simulink model "SkywalkerX8_SensorSuite"  (R2018a)
settings: Solver=FixedStepAuto  StartTime=0.0  StopTime=SkywalkerX8.Sensors.TestProfile.Time(end)  FixedStep=SkywalkerX8.Sensors.TestProfile.Time(2)/100  RelTol=1e-3
undefined symbols (not defined in the file): SkywalkerX8
libraries: sensors x7
settings Model: Creator=David  LastModifiedBy=David

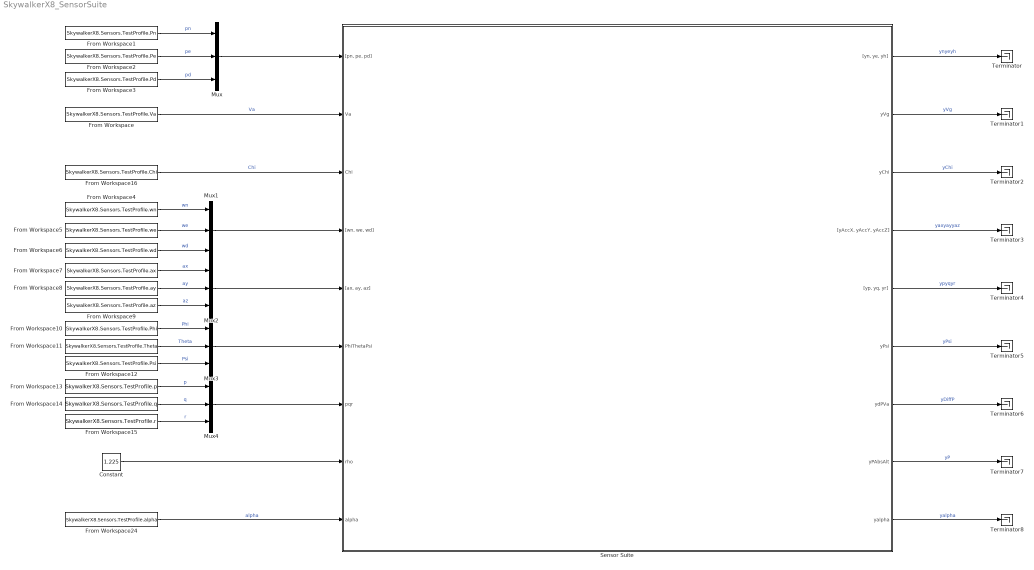
== system SkywalkerX8_SensorSuite ==
  Constant : Constant  Value=1.225
  From Workspace : FromWorkspace  VariableName=SkywalkerX8.Sensors.TestProfile.Va  SampleTime=SkywalkerX8.Sensors.TestProfile.Time(2)  Interpolate=off  OutputAfterFinalValue=Holding final value
  From Workspace1 : FromWorkspace  VariableName=SkywalkerX8.Sensors.TestProfile.Pn  SampleTime=SkywalkerX8.Sensors.TestProfile.Time(2)  Interpolate=off  OutputAfterFinalValue=Holding final value
  From Workspace10 : FromWorkspace  VariableName=SkywalkerX8.Sensors.TestProfile.Phi  SampleTime=SkywalkerX8.Sensors.TestProfile.Time(2)  Interpolate=off  OutputAfterFinalValue=Holding final value
  From Workspace11 : FromWorkspace  VariableName=SkywalkerX8.Sensors.TestProfile.Theta  SampleTime=SkywalkerX8.Sensors.TestProfile.Time(2)  Interpolate=off  OutputAfterFinalValue=Holding final value
  From Workspace12 : FromWorkspace  VariableName=SkywalkerX8.Sensors.TestProfile.Psi  SampleTime=SkywalkerX8.Sensors.TestProfile.Time(2)  Interpolate=off  OutputAfterFinalValue=Holding final value
  From Workspace13 : FromWorkspace  VariableName=SkywalkerX8.Sensors.TestProfile.p  SampleTime=SkywalkerX8.Sensors.TestProfile.Time(2)  Interpolate=off  OutputAfterFinalValue=Holding final value
  From Workspace14 : FromWorkspace  VariableName=SkywalkerX8.Sensors.TestProfile.q  SampleTime=SkywalkerX8.Sensors.TestProfile.Time(2)  Interpolate=off  OutputAfterFinalValue=Holding final value
  From Workspace15 : FromWorkspace  VariableName=SkywalkerX8.Sensors.TestProfile.r  SampleTime=SkywalkerX8.Sensors.TestProfile.Time(2)  Interpolate=off  OutputAfterFinalValue=Holding final value
  From Workspace16 : FromWorkspace  VariableName=SkywalkerX8.Sensors.TestProfile.Chi  SampleTime=SkywalkerX8.Sensors.TestProfile.Time(2)  Interpolate=off  OutputAfterFinalValue=Holding final value
  From Workspace2 : FromWorkspace  VariableName=SkywalkerX8.Sensors.TestProfile.Pe  SampleTime=SkywalkerX8.Sensors.TestProfile.Time(2)  Interpolate=off  OutputAfterFinalValue=Holding final value
  From Workspace24 : FromWorkspace  VariableName=SkywalkerX8.Sensors.TestProfile.alpha  SampleTime=SkywalkerX8.Sensors.TestProfile.Time(2)  Interpolate=off  OutputAfterFinalValue=Holding final value
  From Workspace3 : FromWorkspace  VariableName=SkywalkerX8.Sensors.TestProfile.Pd  SampleTime=SkywalkerX8.Sensors.TestProfile.Time(2)  Interpolate=off  OutputAfterFinalValue=Holding final value
  From Workspace4 : FromWorkspace  VariableName=SkywalkerX8.Sensors.TestProfile.wn  SampleTime=SkywalkerX8.Sensors.TestProfile.Time(2)  Interpolate=off  OutputAfterFinalValue=Holding final value
  From Workspace5 : FromWorkspace  VariableName=SkywalkerX8.Sensors.TestProfile.we  SampleTime=SkywalkerX8.Sensors.TestProfile.Time(2)  Interpolate=off  OutputAfterFinalValue=Holding final value
  From Workspace6 : FromWorkspace  VariableName=SkywalkerX8.Sensors.TestProfile.wd  SampleTime=SkywalkerX8.Sensors.TestProfile.Time(2)  Interpolate=off  OutputAfterFinalValue=Holding final value
  From Workspace7 : FromWorkspace  VariableName=SkywalkerX8.Sensors.TestProfile.ax  SampleTime=SkywalkerX8.Sensors.TestProfile.Time(2)  Interpolate=off  OutputAfterFinalValue=Holding final value
  From Workspace8 : FromWorkspace  VariableName=SkywalkerX8.Sensors.TestProfile.ay  SampleTime=SkywalkerX8.Sensors.TestProfile.Time(2)  Interpolate=off  OutputAfterFinalValue=Holding final value
  From Workspace9 : FromWorkspace  VariableName=SkywalkerX8.Sensors.TestProfile.az  SampleTime=SkywalkerX8.Sensors.TestProfile.Time(2)  Interpolate=off  OutputAfterFinalValue=Holding final value
  Mux{,1..4} (5 alike) : Mux  Inputs=3
  Sensor Suite : Subsystem
      mask Display:
      | image('telemetry.jpg')
      | 
      | color('cyan')
      | 
      | port_label('input', 1, '[p_N, p_E, p_D] (m)', 'texMode', 'On')
      | port_label('input', 2, 'V_a (m/s)', 'texMode', 'On')
      | port_label('input', 3, '\chi (rad)', 'texMode', 'On')
      | port_label('input', 4, '[w_N, w_E, w_D] (m/s)', 'texMode', 'On')
      | port_label('input', 5, '{\bfa_{inertial}} (m/s^2)', 'texMode', 'on')
      | port_label('input', 6, '[\phi, \theta, \psi] (rad)', 'texMode', 'on')
      | port_label('input', 7, '{\bf\omega_b} (rad/s)', 'texMode', 'on')
      | port_label('input', 8, '\rho (kg/m^3)', 'texMode', 'on')
      | port_label('input', 9, '\alpha (rad)', 'texMode', 'on')
      | 
      | port_label('output', 1, '[y_{GPS_N}, y_{GPS_E}, y_{GPS_h}] (m)', 'texMode', 'On')
      | port_label('output', 2, 'y_{GPS_{Vg}} (m/s)', 'texMode', 'On')
      | port_label('output', 3, 'y_{GPS_{\chi}} (rad)', 'texMode', 'On')
      | port_label('output', 4, '[y_{accel_x}, y_{accel_y}, y_{accel_z}] (m/s^2)', 'texMode', 'on')
      | port_label('output', 5, '[y_p, y_q, y_r] (rad/s)', 'texMode', 'on')
      | port_label('output', 6, 'y_{\psi} (rad)', 'texMode', 'on')
      | port_label('output', 7, 'y_{\DeltaP_{V_a}} (Pa)', 'texMode', 'on')
      | port_label('output', 8, 'y_{P_{abs}} (Pa)', 'texMode', 'on')
      | port_label('output', 9, 'y_\alpha (rad)', 'texMode', 'on')
  Terminator{,1..8} (9 alike) : Terminator
  wires:
  Sensor Suite/1("[yn, ye, yh]") -> Terminator/1  "ynyeyh"
  Sensor Suite/2(yVg) -> Terminator1/1  "yVg"
  Sensor Suite/3(yChi) -> Terminator2/1  "yChi"
  Sensor Suite/4("[yAccX, yAccY, yAccZ]") -> Terminator3/1  "yaxyayyaz"
  Sensor Suite/5("[yp, yq, yr]") -> Terminator4/1  "ypyqyr"
  Sensor Suite/6(yPsi) -> Terminator5/1  "yPsi"
  Sensor Suite/7(ydPVa) -> Terminator6/1  "yDiffP"
  Sensor Suite/8(yPAbsAlt) -> Terminator7/1  "yP"
  Mux3/1 -> Sensor Suite/6(PhiThetaPsi)
  Mux/1 -> Sensor Suite/1("[pn, pe, pd]")
  Mux4/1 -> Sensor Suite/7(pqr)
  Mux1/1 -> Sensor Suite/4("[wn, we, wd]")
  From Workspace3/1 -> Mux/3  "pd"
  From Workspace6/1 -> Mux1/3  "wd"
  From Workspace9/1 -> Mux2/3  "az"
  Constant/1 -> Sensor Suite/8(rho)
  From Workspace1/1 -> Mux/1  "pn"
  From Workspace11/1 -> Mux3/2  "Theta"
  From Workspace7/1 -> Mux2/1  "ax"
  From Workspace10/1 -> Mux3/1  "Phi"
  From Workspace4/1 -> Mux1/1  "wn"
  From Workspace8/1 -> Mux2/2  "ay"
  From Workspace12/1 -> Mux3/3  "Psi"
  From Workspace2/1 -> Mux/2  "pe"
  From Workspace14/1 -> Mux4/2  "q"
  From Workspace5/1 -> Mux1/2  "we"
  From Workspace/1 -> Sensor Suite/2(Va)  "Va"
  From Workspace15/1 -> Mux4/3  "r"
  Mux2/1 -> Sensor Suite/5("[ax, ay, az]")
  From Workspace13/1 -> Mux4/1  "p"
  From Workspace24/1 -> Sensor Suite/9(alpha)  "alpha"
  Sensor Suite/9(yalpha) -> Terminator8/1  "yalpha"
  From Workspace16/1 -> Sensor Suite/3(Chi)  "Chi"

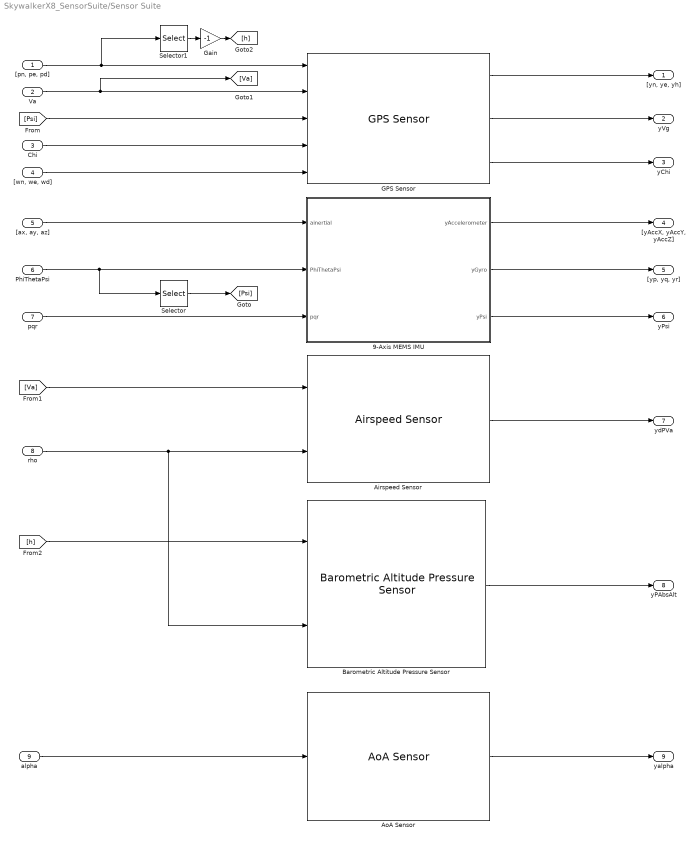
== system SkywalkerX8_SensorSuite/Sensor Suite ==
  "[pn, pe, pd]" : Inport
  Va : Inport  Port=2
  Chi : Inport  Port=3
  "[wn, we, wd]" : Inport  Port=4
  "[ax, ay, az]" : Inport  Port=5
  PhiThetaPsi : Inport  Port=6
  pqr : Inport  Port=7
  rho : Inport  Port=8
  alpha : Inport  Port=9
  9-Axis MEMS IMU : Subsystem
      mask Display:
      | image('VNAV_IMU.jpg')
      | 
      | color('green')
      | 
      | port_label('input', 1, '{\bfa_{inertial}} (m/s^2)', 'texMode', 'on')
      | port_label('input', 2, '[\phi, \theta, \psi] (rad)', 'texMode', 'on')
      | port_label('input', 3, '{\bf\omega_b} (rad/s)', 'texMode', 'on')
      | 
      | port_label('output', 1, '[y_{accel_x}, y_{accel_y}, y_{accel_z}] (m/s^2)', 'texMode', 'on')
      | port_label('output', 2, '[y_p, y_q, y_r] (rad/s)', 'texMode', 'on')
      | port_label('output', 3, 'y_{\psi} (rad)', 'texMode', 'on')
  Airspeed Sensor : sensors/Airspeed Sensor  SampleTime=SkywalkerX8.Sensors.AirspeedPressure.SampleTime  diffPressureStdDev=SkywalkerX8.Sensors.AirspeedPressure.StdDev  diffPressureBandwidthHz=SkywalkerX8.Sensors.AirspeedPressure.BandwidthHz  diffPressureInit=SkywalkerX8.Sensors.AirspeedPressure.InitialCondition  diffPressureUpperSaturation=SkywalkerX8.Sensors.AirspeedPressure.UpperSat  diffPressureLowerSaturation=SkywalkerX8.Sensors.AirspeedPressure.LowerSat  diffPressureResolution=SkywalkerX8.Sensors.AirspeedPressure.Resolution
  AoA Sensor : sensors/AoA Sensor  SampleTime=SkywalkerX8.Sensors.AoA.SampleTime  alphaStdDev=SkywalkerX8.Sensors.AoA.StdDev  alphaBandwidthHz=SkywalkerX8.Sensors.AoA.BandwidthHz  alphaInit=SkywalkerX8.Sensors.AoA.InitialCondition  alphaUpperSaturation=SkywalkerX8.Sensors.AoA.UpperSat  alphaLowerSaturation=SkywalkerX8.Sensors.AoA.LowerSat  alphaResolution=SkywalkerX8.Sensors.AoA.Resolution
  Barometric Altitude Pressure Sensor : sensors/Barometric Altitude Pressure Sensor  g=SkywalkerX8.System.Gravity  SampleTime=SkywalkerX8.Sensors.AltitudePressure.SampleTime  absPressureStdDev=SkywalkerX8.Sensors.AltitudePressure.StdDev  absPressureBandwidthHz=SkywalkerX8.Sensors.AltitudePressure.BandwidthHz  absPressureInit=SkywalkerX8.Sensors.AltitudePressure.InitialCondition  absPressureUpperSaturation=SkywalkerX8.Sensors.AltitudePressure.UpperSat  absPressureLowerSaturation=SkywalkerX8.Sensors.AltitudePressure.LowerSat  absPressureResolution=SkywalkerX8.Sensors.AltitudePressure.Resolution
  GPS Sensor : sensors/GPS Sensor  SampleTime=SkywalkerX8.Sensors.GPS.SampleTime  pnInit=SkywalkerX8.Sensors.GPS.pnInit  peInit=SkywalkerX8.Sensors.GPS.peInit  pdInit=SkywalkerX8.Sensors.GPS.pdInit  VgInit=SkywalkerX8.Sensors.GPS.VgInit  ChiInit=SkywalkerX8.Sensors.GPS.ChiInit  GPSNStdDev=SkywalkerX8.Sensors.GPS.North.StdDev  OneOverkGPSN=SkywalkerX8.Sensors.GPS.North.TimeConstant  GPSEStdDev=SkywalkerX8.Sensors.GPS.East.StdDev  OneOverkGPSE=SkywalkerX8.Sensors.GPS.East.TimeConstant  GPSAltStdDev=SkywalkerX8.Sensors.GPS.Alt.StdDev  OneOverkGPSAlt=SkywalkerX8.Sensors.GPS.Alt.TimeConstant  GPSVStdDev=SkywalkerX8.Sensors.GPS.Velocity.StdDev
  Gain : Gain  Gain=-1
  Selector : Selector  InputPortWidth=3  IndexOptions=Index vector (dialog)  Indices=3  OutputSizes=1
  Selector1 : Selector  InputPortWidth=3  IndexOptions=Index vector (dialog)  Indices=3  OutputSizes=1
  "[yn, ye, yh]" : Outport
  yVg : Outport  Port=2
  yChi : Outport  Port=3
  "[yAccX, yAccY, yAccZ]" : Outport  Port=4
  "[yp, yq, yr]" : Outport  Port=5
  yPsi : Outport  Port=6
  ydPVa : Outport  Port=7
  yPAbsAlt : Outport  Port=8
  yalpha : Outport  Port=9
  wires:
  "[pn, pe, pd]"/1 -> GPS Sensor/1, Selector1/1
  Va/1 -> [Va], GPS Sensor/2
  PhiThetaPsi/1 -> 9-Axis MEMS IMU/2(PhiThetaPsi), Selector/1
  Airspeed Sensor/1 -> ydPVa/1
  [Psi] -> GPS Sensor/3
  Selector1/1 -> Gain/1
  rho/1 -> Barometric Altitude Pressure Sensor/2, Airspeed Sensor/2
  GPS Sensor/3 -> yChi/1
  Selector/1 -> [Psi]
  [h] -> Barometric Altitude Pressure Sensor/1
  9-Axis MEMS IMU/3(yPsi) -> yPsi/1
  [Va] -> Airspeed Sensor/1
  pqr/1 -> 9-Axis MEMS IMU/3(pqr)
  9-Axis MEMS IMU/2(yGyro) -> "[yp, yq, yr]"/1
  "[wn, we, wd]"/1 -> GPS Sensor/5
  Barometric Altitude Pressure Sensor/1 -> yPAbsAlt/1
  GPS Sensor/1 -> "[yn, ye, yh]"/1
  Gain/1 -> [h]
  GPS Sensor/2 -> yVg/1
  "[ax, ay, az]"/1 -> 9-Axis MEMS IMU/1(ainertial)
  9-Axis MEMS IMU/1(yAccelerometer) -> "[yAccX, yAccY, yAccZ]"/1
  AoA Sensor/1 -> yalpha/1
  alpha/1 -> AoA Sensor/1
  Chi/1 -> GPS Sensor/4

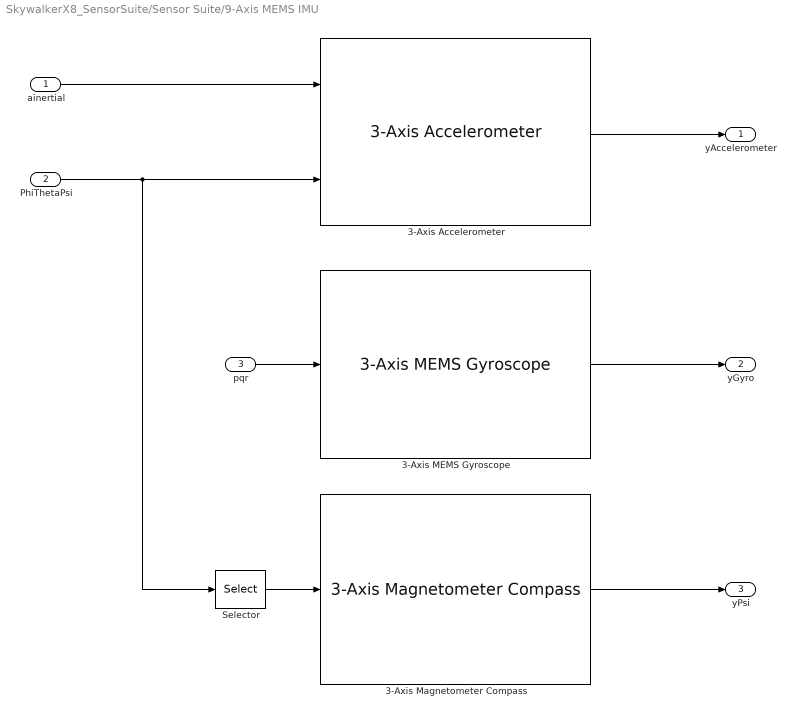
== system SkywalkerX8_SensorSuite/Sensor Suite/9-Axis MEMS IMU ==
  ainertial : Inport
  PhiThetaPsi : Inport  Port=2
  pqr : Inport  Port=3
  3-Axis Accelerometer : sensors/3-Axis Accelerometer  g=SkywalkerX8.System.Gravity  SampleTime=SkywalkerX8.Sensors.IMU.Accelerometer.SampleTime  accelXNoiseDensity=SkywalkerX8.Sensors.IMU.Accelerometer.X.NoiseDensity  accelYNoiseDensity=SkywalkerX8.Sensors.IMU.Accelerometer.Y.NoiseDensity  accelZNoiseDensity=SkywalkerX8.Sensors.IMU.Accelerometer.Z.NoiseDensity  accelXBandwidthHz=SkywalkerX8.Sensors.IMU.Accelerometer.X.BandwidthHz  accelYBandwidthHz=SkywalkerX8.Sensors.IMU.Accelerometer.Y.BandwidthHz  accelZBandwidthHz=SkywalkerX8.Sensors.IMU.Accelerometer.Z.BandwidthHz  accelXInit=SkywalkerX8.Sensors.IMU.Accelerometer.X.InitialCondition  accelYInit=SkywalkerX8.Sensors.IMU.Accelerometer.Y.InitialCondition  accelZInit=SkywalkerX8.Sensors.IMU.Accelerometer.Z.InitialCondition  accelXUpperSaturation=SkywalkerX8.Sensors.IMU.Accelerometer.X.UpperSat  accelXLowerSaturation=SkywalkerX8.Sensors.IMU.Accelerometer.X.LowerSat  accelYUpperSaturation=SkywalkerX8.Sensors.IMU.Accelerometer.Y.UpperSat  accelYLowerSaturation=SkywalkerX8.Sensors.IMU.Accelerometer.Y.LowerSat  accelZUpperSaturation=SkywalkerX8.Sensors.IMU.Accelerometer.Z.UpperSat  accelZLowerSaturation=SkywalkerX8.Sensors.IMU.Accelerometer.Z.LowerSat  accelXResolution=SkywalkerX8.Sensors.IMU.Accelerometer.X.Resolution  accelYResolution=SkywalkerX8.Sensors.IMU.Accelerometer.Y.Resolution  accelZResolution=SkywalkerX8.Sensors.IMU.Accelerometer.Z.Resolution
  3-Axis MEMS Gyroscope : sensors/3-Axis MEMS Gyroscope  SampleTime=SkywalkerX8.Sensors.IMU.Gyroscope.SampleTime  gyroXNoiseDensity=SkywalkerX8.Sensors.IMU.Gyroscope.X.NoiseDensity  gyroYNoiseDensity=SkywalkerX8.Sensors.IMU.Gyroscope.Y.NoiseDensity  gyroZNoiseDensity=SkywalkerX8.Sensors.IMU.Gyroscope.Z.NoiseDensity  gyroXBandwidthHz=SkywalkerX8.Sensors.IMU.Gyroscope.X.BandwidthHz  gyroYBandwidthHz=SkywalkerX8.Sensors.IMU.Gyroscope.Y.BandwidthHz  gyroZBandwidthHz=SkywalkerX8.Sensors.IMU.Gyroscope.Z.BandwidthHz  gyroXInit=SkywalkerX8.Sensors.IMU.Gyroscope.X.InitialCondition  gyroYInit=SkywalkerX8.Sensors.IMU.Gyroscope.Y.InitialCondition  gyroZInit=SkywalkerX8.Sensors.IMU.Gyroscope.Z.InitialCondition  gyroXUpperSaturation=SkywalkerX8.Sensors.IMU.Gyroscope.X.UpperSat  gyroXLowerSaturation=SkywalkerX8.Sensors.IMU.Gyroscope.X.LowerSat  gyroYUpperSaturation=SkywalkerX8.Sensors.IMU.Gyroscope.Y.UpperSat  gyroYLowerSaturation=SkywalkerX8.Sensors.IMU.Gyroscope.Y.LowerSat  gyroZUpperSaturation=SkywalkerX8.Sensors.IMU.Gyroscope.Z.UpperSat  gyroZLowerSaturation=SkywalkerX8.Sensors.IMU.Gyroscope.Z.LowerSat  gyroXResolution=SkywalkerX8.Sensors.IMU.Gyroscope.X.Resolution  gyroYResolution=SkywalkerX8.Sensors.IMU.Gyroscope.Y.Resolution  gyroZResolution=SkywalkerX8.Sensors.IMU.Gyroscope.Z.Resolution
  3-Axis Magnetometer Compass : sensors/3-Axis Magnetometer Compass  SampleTime=SkywalkerX8.Sensors.IMU.Compass.SampleTime  headingNoiseDensity=SkywalkerX8.Sensors.IMU.Compass.NoiseDensity  headingBandwidthHz=SkywalkerX8.Sensors.IMU.Compass.BandwidthHz  headingInit=SkywalkerX8.Sensors.IMU.Compass.InitialCondition  headingUpperSaturation=SkywalkerX8.Sensors.IMU.Compass.UpperSat  headingLowerSaturation=SkywalkerX8.Sensors.IMU.Compass.LowerSat  headingResolution=SkywalkerX8.Sensors.IMU.Compass.Resolution
  Selector : Selector  InputPortWidth=3  IndexOptions=Index vector (dialog)  Indices=3  OutputSizes=1
  yAccelerometer : Outport
  yGyro : Outport  Port=2
  yPsi : Outport  Port=3
  wires:
  ainertial/1 -> 3-Axis Accelerometer/1
  PhiThetaPsi/1 -> 3-Axis Accelerometer/2, Selector/1
  Selector/1 -> 3-Axis Magnetometer Compass/1
  pqr/1 -> 3-Axis MEMS Gyroscope/1
  3-Axis MEMS Gyroscope/1 -> yGyro/1
  3-Axis Accelerometer/1 -> yAccelerometer/1
  3-Axis Magnetometer Compass/1 -> yPsi/1
